simulink model "LQG_model_newone"  (R2023a)
settings: Solver=FixedStepDiscrete  StartTime=0.0  StopTime=2  FixedStep=Ts  RelTol=1e-3
values from neighbouring files (symbols this model uses):
  Ad = expm(A*Ts)    [Assignment_M32.m]
  C1 = [0,1,0,0,0;0,0,0,0,1]    [Assignment_M32.m]
  doubleBd = double(Bd)    [Assignment_M32.m]
  K_fb = Klqr(:,1:length(Ad))    [Assignment_M32.m]
  K_I = Klqr(:,length(Ad)+1:end)*20    [Assignment_M32.m]
  sigma2_phi2 = calcVariance(0.02, 0.997)    [Assignment_M32.m]
  sigma2_Te = calcVariance(0.1, 0.997)    [Assignment_M32.m]
  sigma2_va = calcVariance(0.3, 0.997)    [Assignment_M32.m]
  sigma2_w2 = calcVariance(0.01, 0.997)    [Assignment_M32.m]
  Ts = 0.001    [Assignment_M32.m]
  x0 = [0 0 0 0 0]'    [Assignment_M32.m]
undefined symbols (not defined in the file or in its folder): C1_I, DiscIntNeverNeededParam, L_kalman, sigbuilder_block
settings Model: Creator=Renata  LastModifiedBy=meng_fanze
settings SolverCC: AlgebraicLoopSolver=TrustRegion
settings DataIOCC: ReturnWorkspaceOutputs=off
settings DebuggingCC: UnconnectedInputMsg=warning  UnconnectedOutputMsg=warning  UnconnectedLineMsg=warning  ArithmeticOperatorsInVariantConditions=warning
settings ModelReferenceCC: EnableRefExpFcnMdlSchedulingChecks=on
settings SFSimCC: CustomCodeUndefinedFunction=UseInterfaceOnly

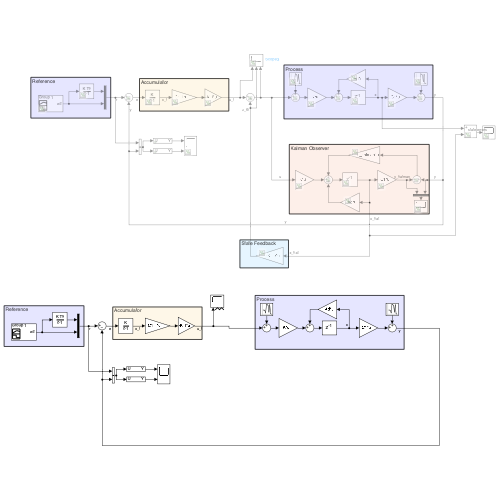
[thumbnail: Simulink's stored preview of the top-level diagram]
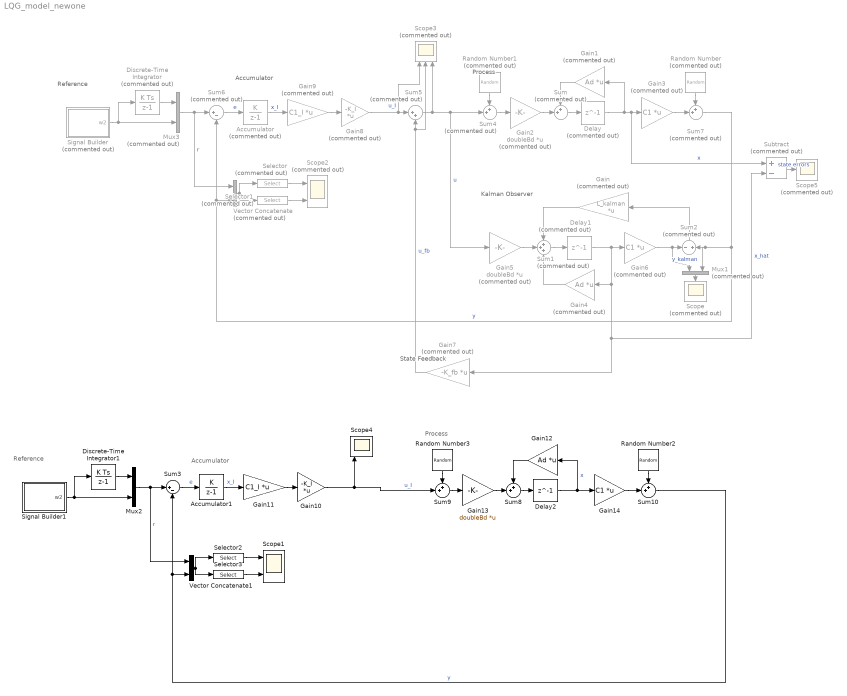
== system LQG_model_newone ==
  note: Reference
  note: State Feedback
  note: Accumulator
  note: Kalman Observer
  note: Process
  note: Reference
  note: Accumulator
  note: Process
  Accumulator : DiscreteIntegrator  Commented=on  IntegratorMethod=Accumulation: Forward Euler  SampleTime=-1  ICPrevOutput=DiscIntNeverNeededParam  ICPrevScaledInput=DiscIntNeverNeededParam
  Accumulator1 : DiscreteIntegrator  IntegratorMethod=Accumulation: Forward Euler  SampleTime=-1  ICPrevOutput=DiscIntNeverNeededParam  ICPrevScaledInput=DiscIntNeverNeededParam
  Delay : Delay  Commented=on  DelayLength=1  InitialCondition=x0
  Delay1 : Delay  Commented=on  DelayLength=1
  Delay2 : Delay  DelayLength=1  InitialCondition=x0
  Discrete-Time Integrator : DiscreteIntegrator  Commented=on  SampleTime=-1  ICPrevOutput=DiscIntNeverNeededParam  ICPrevScaledInput=DiscIntNeverNeededParam
  Discrete-Time Integrator1 : DiscreteIntegrator  SampleTime=-1  ICPrevOutput=DiscIntNeverNeededParam  ICPrevScaledInput=DiscIntNeverNeededParam
  Gain : Gain  Commented=on  Gain=L_kalman  Multiplication=Matrix(K*u)
  Gain1 : Gain  Commented=on  Gain=Ad  Multiplication=Matrix(K*u)
  Gain10 : Gain  Gain=-K_I  Multiplication=Matrix(K*u)
  Gain11 : Gain  Gain=C1_I  Multiplication=Matrix(K*u)
  Gain12 : Gain  Gain=Ad  Multiplication=Matrix(K*u)
  Gain13 : Gain  Gain=doubleBd  Multiplication=Matrix(K*u)
  Gain14 : Gain  Gain=C1  Multiplication=Matrix(K*u)
  Gain2 : Gain  Commented=on  Gain=doubleBd  Multiplication=Matrix(K*u)
  Gain3 : Gain  Commented=on  Gain=C1  Multiplication=Matrix(K*u)
  Gain4 : Gain  Commented=on  Gain=Ad  Multiplication=Matrix(K*u)
  Gain5 : Gain  Commented=on  Gain=doubleBd  Multiplication=Matrix(K*u)
  Gain6 : Gain  Commented=on  Gain=C1  Multiplication=Matrix(K*u)
  Gain7 : Gain  Commented=on  Gain=-K_fb  Multiplication=Matrix(K*u)
  Gain8 : Gain  Commented=on  Gain=-K_I  Multiplication=Matrix(K*u)
  Gain9 : Gain  Commented=on  Gain=C1_I  Multiplication=Matrix(K*u)
  Mux1 : Mux  Commented=on  Inputs=2
  Mux2 : Mux  Inputs=2
  Mux3 : Mux  Commented=on  Inputs=2
  Random Number : RandomNumber  Commented=on  Variance=[sigma2_phi2 sigma2_w2]  SampleTime=Ts
  Random Number1 : RandomNumber  Commented=on  Variance=[sigma2_va,sigma2_Te]  SampleTime=Ts
  Random Number2 : RandomNumber  Variance=[sigma2_phi2 sigma2_w2]  SampleTime=Ts
  Random Number3 : RandomNumber  Variance=[sigma2_va,sigma2_Te]  SampleTime=Ts
  Scope : Scope  Commented=on
  Scope1 : Scope  NumInputPorts=2
  Scope2 : Scope  Commented=on  NumInputPorts=2
  Scope3 : Scope  Commented=on  NumInputPorts=3
  Scope4 : Scope  NumInputPorts=3
  Scope5 : Scope  Commented=on
  Selector : Selector  Commented=on  InputPortWidth=4  IndexOptions=Index vector (dialog)  Indices=[1 3]  OutputSizes=1
  Selector1 : Selector  Commented=on  InputPortWidth=4  IndexOptions=Index vector (dialog)  Indices=[2 4]  OutputSizes=1
  Selector2 : Selector  InputPortWidth=4  IndexOptions=Index vector (dialog)  Indices=[1 3]  OutputSizes=1
  Selector3 : Selector  InputPortWidth=4  IndexOptions=Index vector (dialog)  Indices=[2 4]  OutputSizes=1
  Signal Builder : Subsystem  Tag=STV Subsys  Commented=on  LoadFcn=sigbuilder_block('load');  StartFcn=sigbuilder_block('start');  StopFcn=sigbuilder_block('stop');  ClipboardFcn=sigbuilder_block('clipboard');  mask(Sigbuilder block){tuvar=[0:10]}
      mask help: Simulink:masks:SigbuilderBlock_MD
      mask init:
      | if ~strcmp(get_param(bdroot(gcbh),'SimulationStatus'),'stopped') tuvar = sigbuilder_block('maskInit'); end
      settings: CopyFcn=sigbuilder_block('copy');  DeleteFcn=sigbuilder_block('delete');  ModelCloseFcn=sigbuilder_block('modelClose');  PreSaveFcn=sigbuilder_block('preSave');  PauseFcn=sigbuilder_block('pause');  ContinueFcn=sigbuilder_block('continue');  NameChangeFcn=sigbuilder_block('namechange');  OpenFcn=sigbuilder_block('open',[367.8 74.4 682.2 467.4 ]);  CloseFcn=sigbuilder_block('close');
      mask Display: plot(0, 0, 100, 100,[2, 2, 32, 32, 2], [68, 8, 8, 68, 68],[32, 2], [38, 38], [32, 19, 2],[53, 60, 44], [32, 17, 17, 2],[16, 16, 31, 31]);txt = getActiveGroup(gcbh);text(2, 100, txt,'verticalAlignment', 'top');
  Signal Builder1 : Subsystem  Tag=STV Subsys  LoadFcn=sigbuilder_block('load');  StartFcn=sigbuilder_block('start');  StopFcn=sigbuilder_block('stop');  ClipboardFcn=sigbuilder_block('clipboard');  mask(Sigbuilder block){tuvar=[0:10]}
      mask help: Simulink:masks:SigbuilderBlock_MD
      mask init:
      | if ~strcmp(get_param(bdroot(gcbh),'SimulationStatus'),'stopped') tuvar = sigbuilder_block('maskInit'); end
      settings: CopyFcn=sigbuilder_block('copy');  DeleteFcn=sigbuilder_block('delete');  ModelCloseFcn=sigbuilder_block('modelClose');  PreSaveFcn=sigbuilder_block('preSave');  PauseFcn=sigbuilder_block('pause');  ContinueFcn=sigbuilder_block('continue');  NameChangeFcn=sigbuilder_block('namechange');  OpenFcn=sigbuilder_block('open',[367.8 74.4 682.2 467.4 ]);  CloseFcn=sigbuilder_block('close');
      mask Display: plot(0, 0, 100, 100,[2, 2, 32, 32, 2], [68, 8, 8, 68, 68],[32, 2], [38, 38], [32, 19, 2],[53, 60, 44], [32, 17, 17, 2],[16, 16, 31, 31]);txt = getActiveGroup(gcbh);text(2, 100, txt,'verticalAlignment', 'top');
  Subtract : Sum  Commented=on  Inputs=+-
  Sum : Sum  Commented=on  Inputs=++|
  Sum1 : Sum  Commented=on  Inputs=+++
  Sum10 : Sum  Inputs=++|
  Sum2 : Sum  Commented=on  Inputs=-|+
  Sum3 : Sum  Inputs=|+-
  Sum4 : Sum  Commented=on  Inputs=++|
  Sum5 : Sum  Commented=on  Inputs=|++
  Sum6 : Sum  Commented=on  Inputs=|+-
  Sum7 : Sum  Commented=on  Inputs=++|
  Sum8 : Sum  Inputs=++|
  Sum9 : Sum  Inputs=++|
  Vector Concatenate : Concatenate  Commented=on
  Vector Concatenate1 : Concatenate
  wires:
  Delay/1 -> Subtract/1, Gain3/1, Gain1/1  "x"
  Sum/1 -> Delay/1
  Gain5/1 -> Sum1/2
  Delay1/1 -> Gain6/1, Gain7/1, Subtract/2, Gain4/1  "x_hat"
  Gain4/1 -> Sum1/3
  Sum1/1 -> Delay1/1
  Gain6/1 -> Mux1/1, Sum2/1  "y_kalman"
  Sum7/1 -> Mux1/2, Sum2/2, Sum6/2, Vector Concatenate/2  "y"
  Sum4/1 -> Gain2/1
  Gain7/1 -> Scope3/2, Sum5/2  "u_fb"
  Sum2/1 -> Gain/1
  Gain/1 -> Sum1/1
  Sum5/1 -> Sum4/2, Gain5/1, Scope3/3  "u"
  Gain8/1 -> Sum5/1, Scope3/1  "u_I"
  Sum6/1 -> Accumulator/1  "e"
  Accumulator/1 -> Gain9/1  "x_I"
  Mux1/1 -> Scope/1
  Subtract/1 -> Scope5/1  "state errors"
  Mux3/1 -> Vector Concatenate/1, Sum6/1  "r"
  Signal Builder/1(w2) -> Discrete-Time Integrator/1, Mux3/2
  Discrete-Time Integrator/1 -> Mux3/1
  Selector/1 -> Scope2/1
  Vector Concatenate/1 -> Selector/1, Selector1/1
  Selector1/1 -> Scope2/2
  Gain9/1 -> Gain8/1
  Gain2/1 -> Sum/2
  Gain1/1 -> Sum/1
  Gain3/1 -> Sum7/2
  Random Number/1 -> Sum7/1
  Random Number1/1 -> Sum4/1
  Selector3/1 -> Scope1/2
  Signal Builder1/1(w2) -> Discrete-Time Integrator1/1, Mux2/2
  Sum3/1 -> Accumulator1/1  "e"
  Selector2/1 -> Scope1/1
  Gain11/1 -> Gain10/1
  Discrete-Time Integrator1/1 -> Mux2/1
  Mux2/1 -> Vector Concatenate1/1, Sum3/1  "r"
  Vector Concatenate1/1 -> Selector2/1, Selector3/1
  Accumulator1/1 -> Gain11/1  "x_I"
  Delay2/1 -> Gain14/1, Gain12/1  "x"
  Sum8/1 -> Delay2/1
  Gain12/1 -> Sum8/1
  Random Number2/1 -> Sum10/1
  Sum9/1 -> Gain13/1
  Gain13/1 -> Sum8/2
  Random Number3/1 -> Sum9/1
  Gain14/1 -> Sum10/2
  Gain10/1 -> Scope4/1, Sum9/2  "u_I"
  Sum10/1 -> Vector Concatenate1/2, Sum3/2  "y"

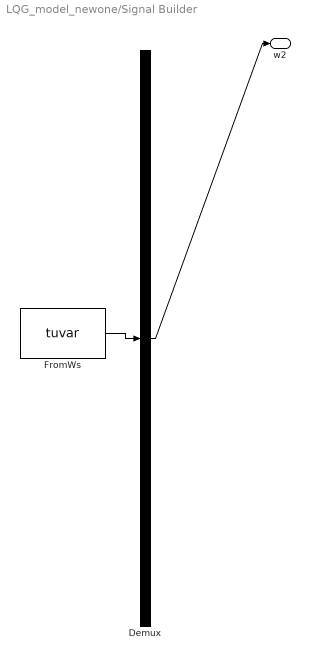
== system LQG_model_newone/Signal Builder ==
  Demux : Demux  Tag=STV Demux  Outputs=1
      settings: DisplayOption=none
  FromWs : FromWorkspace  Tag=STV FromWs  VariableName=tuvar
      SigBuilderData=|
      | common.afterFinalStr = 'Extrapolate'
      | common.sampleTime = 0
      | dataSet.timeRange = [0 10]
      | dataSet.name = 'Group 1'
      | sbobj.Groups.Name = 'Group 1'
      | sbobj.Groups.Signals.Name = 'w2'
      | sbobj.Groups.Signals.XData = [0 0.5 0.5 10]
      | sbobj.Groups.Signals.YData = [10 10 100 100]
  w2 : Outport  Tag=STV Outport  VectorParamsAs1DForOutWhenUnconnected=off
  wires:
  FromWs/1 -> Demux/1
  Demux/1 -> w2/1

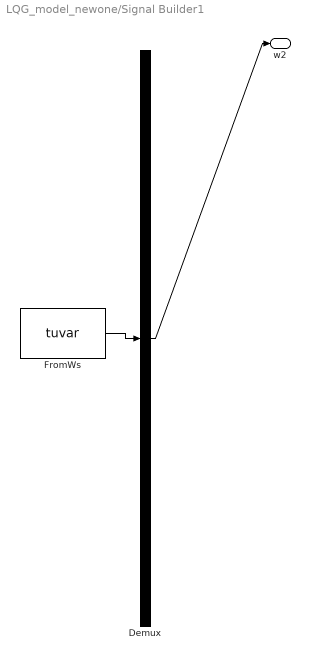
== system LQG_model_newone/Signal Builder1 ==
  Demux : Demux  Tag=STV Demux  Outputs=1
      settings: DisplayOption=none
  FromWs : FromWorkspace  Tag=STV FromWs  VariableName=tuvar
      SigBuilderData=|
      | common.afterFinalStr = 'Extrapolate'
      | common.sampleTime = 0
      | dataSet.timeRange = [0 10]
      | dataSet.name = 'Group 1'
      | sbobj.Groups.Name = 'Group 1'
      | sbobj.Groups.Signals.Name = 'w2'
      | sbobj.Groups.Signals.XData = [0 0.5 0.5 10]
      | sbobj.Groups.Signals.YData = [10 10 100 100]
  w2 : Outport  Tag=STV Outport  VectorParamsAs1DForOutWhenUnconnected=off
  wires:
  FromWs/1 -> Demux/1
  Demux/1 -> w2/1
